simulink model "auv_backstepping2017"  (R2017b)
settings: Solver=VariableStepAuto  StartTime=0.0  StopTime=300.00  RelTol=1e-3
libraries: simulink x1
settings Model: Creator=aditya-ubuntu  LastModifiedBy=Aditya Ravi
settings SFSimCC: SimUseLocalCustomCode=on
settings RTWCC: RTWUseLocalCustomCode=on

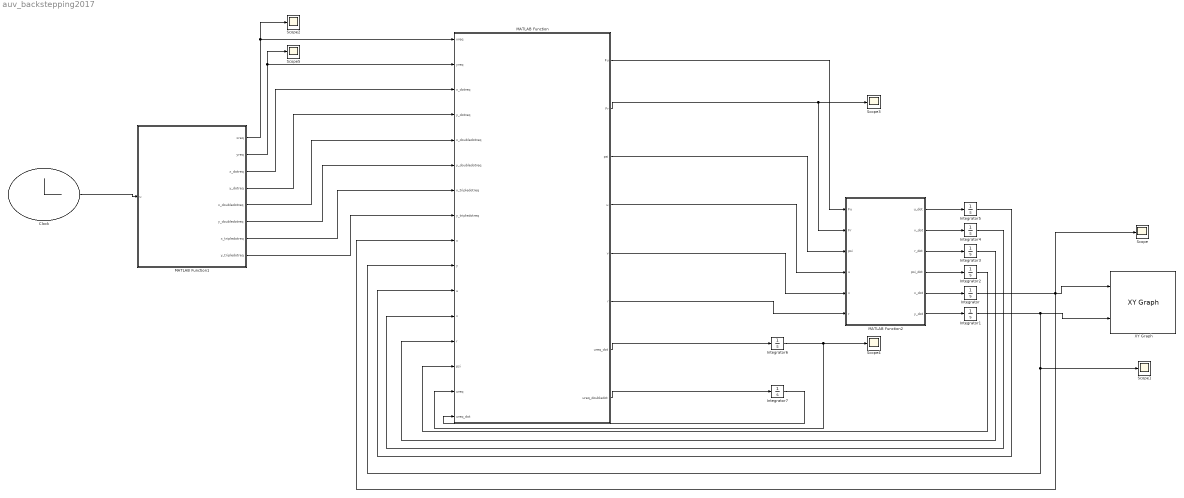
== system auv_backstepping2017 ==
  Clock : Clock
      settings: Decimation=30
  Integrator{,1..5,7} (7 alike) : Integrator
  Integrator6 : Integrator  InitialCondition=0.001  LimitOutput=on  UpperSaturationLimit=+10  LowerSaturationLimit=-10
  MATLAB Function : MATLAB Function  TreatAsAtomicUnit=on
  MATLAB Function1 : MATLAB Function  TreatAsAtomicUnit=on
  MATLAB Function2 : MATLAB Function  TreatAsAtomicUnit=on
  Scope{,1..5} (6 alike) : Scope
  XY Graph : simulink/Sinks/XY Graph  xmin=-20  xmax=20  ymin=-20  ymax=20  st=-1
  wires:
  MATLAB Function/1(Fu) -> MATLAB Function2/1(Fu)
  MATLAB Function/2(Fr) -> MATLAB Function2/2(Fr), Scope3/1
  MATLAB Function2/6(y_dot) -> Integrator1/1
  MATLAB Function2/5(x_dot) -> Integrator/1
  MATLAB Function2/4(psi_dot) -> Integrator2/1
  MATLAB Function2/3(r_dot) -> Integrator3/1
  MATLAB Function2/2(v_dot) -> Integrator4/1
  MATLAB Function2/1(u_dot) -> Integrator5/1
  Integrator/1 -> XY Graph/1, MATLAB Function/9(x), Scope/1
  Integrator1/1 -> XY Graph/2, MATLAB Function/10(y), Scope1/1
  Integrator6/1 -> MATLAB Function/15(ureq), Scope4/1
  Integrator5/1 -> MATLAB Function/11("u ")
  Integrator3/1 -> MATLAB Function/13("r ")
  Integrator2/1 -> MATLAB Function/14("psi ")
  MATLAB Function/4(u) -> MATLAB Function2/4(u)
  MATLAB Function/5(v) -> MATLAB Function2/5(v)
  MATLAB Function/6(r) -> MATLAB Function2/6(r)
  Integrator4/1 -> MATLAB Function/12("v ")
  MATLAB Function/3(psi) -> MATLAB Function2/3(psi)
  MATLAB Function/8(ureq_doubledot) -> Integrator7/1
  MATLAB Function/7(ureq_dot) -> Integrator6/1
  Integrator7/1 -> MATLAB Function/16("ureq_dot ")
  Clock/1 -> MATLAB Function1/1(u)
  MATLAB Function1/3(x_dotreq) -> MATLAB Function/3(x_dotreq)
  MATLAB Function1/4(y_dotreq) -> MATLAB Function/4(y_dotreq)
  MATLAB Function1/5(x_doubledotreq) -> MATLAB Function/5(x_doubledotreq)
  MATLAB Function1/6(y_doubledotreq) -> MATLAB Function/6(y_doubledotreq)
  MATLAB Function1/7(x_tripledotreq) -> MATLAB Function/7(x_tripledotreq)
  MATLAB Function1/8(y_tripledotreq) -> MATLAB Function/8(y_tripledotreq)
  MATLAB Function1/2(yreq) -> Scope5/1, MATLAB Function/2(yreq)
  MATLAB Function1/1(xreq) -> MATLAB Function/1(xreq), Scope2/1

== matlab function auv_backstepping2017/MATLAB Function1 ==
  data: xreq output; yreq output; u input; x_dotreq output; y_dotreq output; x_doubledotreq output; y_doubledotreq output; x_tripledotreq output; y_tripledotreq output
function [xreq,yreq,x_dotreq,y_dotreq,x_doubledotreq,y_doubledotreq,x_tripledotreq,y_tripledotreq] = fcn(u)

a = 10;
b = 0.1;

xreq = a*sin(b*u);
yreq = a*cos(b*u);

x_dotreq = a*b*cos(b*u);
y_dotreq = -a*b*sin(b*u);

x_doubledotreq = -a*b*b*sin(b*u);
y_doubledotreq = -a*b*b*cos(b*u);

x_tripledotreq = -a*b*b*b*cos(b*u);
y_tripledotreq = a*b*b*b*sin(b*u);

== matlab function auv_backstepping2017/MATLAB Function ==
  data: xreq input; yreq input; Fu output; x_dotreq input; y_dotreq input; x_doubledotreq input; y_doubledotreq input; x_tripledotreq input; y_tripledotreq input; x input; y input; u input; v input; r input; psi input; Fr output; psi output; u output; v output; r output; ureq_dot output; ureq_doubledot output; ureq input; ureq_dot input
function [Fu,Fr,psi,u,v,r,ureq_dot,ureq_doubledot] = fcn(xreq, yreq, x_dotreq, y_dotreq,x_doubledotreq,y_doubledotreq,x_tripledotreq,y_tripledotreq,x,y,u,v,r,psi,ureq,ureq_dot)

% constants 
mass= 185.0;                                                % Mass kg
Iz = 50.0;                                                  % Rotational inertia kg-m2
Xu = -30.0;                                                 % added mass kg
Yv = -90.0;                                                 % added mass kg
Nr = -30.0;                                                 % added mass kg
m = [(mass-Xu); (mass-Yv); (Iz-Nr)];                        % combined inertia and added mass terms
onebym = [1.0/(mass-Xu); 1.0/(mass-Yv); 1.0/(Iz-Nr)];       % one by combined inertia and added mass terms
d = [70.0; 100.0; 50.0];                                    % linear drag [surge, sway, yaw]

vp = sqrt(x_dotreq^2 + y_dotreq^2);
vp_dot = ((x_dotreq*x_doubledotreq)+ (y_dotreq*y_doubledotreq))/vp;
beta = atan2(y_dotreq,x_dotreq);
while(beta<0)
            beta = beta + 2*pi;
end        
while(beta>6.28)
            beta = beta - 2*pi;
end

beta_dot = ((x_dotreq*y_doubledotreq) - (y_dotreq*x_doubledotreq))/(vp^2);

if(beta_dot<=0)    
         if(ureq>=0.1)
             ureq = 0.1;
             vreq = 0;
             rreq = 0;
             psireq = beta;
             disp("ureq is equal to vp");       
         else 
             vreq = sqrt((vp*vp) - (ureq*ureq));
             mu = atan2(vreq,ureq);
             while(mu<0)
                mu = mu + 2*pi;
             end 
             while(mu>6.28)
                mu = mu - 2*pi;
             end
             psireq = beta - mu;
             rreq = beta_dot - ((ureq*vp_dot - ureq_dot*vp)/(vp*abs(vreq)));
         end 
else
         if(ureq>=0.1)
             ureq = 0.1;
             vreq = 0;
             rreq = 0;
             psireq = beta;
             disp("error");       
         else
             vreq = -sqrt((vp*vp) - (ureq*ureq));
             mu = atan2(vreq,ureq);
             while(mu<0)
                mu = mu + 2*pi;
             end    
             while(mu>6.28)
                 mu = mu - 2*pi;
             end
             psireq = beta + mu;
             rreq = beta_dot + ((ureq*vp_dot - ureq_dot*vp)/(vp*abs(vreq)));
         end 
end

beta_doubledot = ((x_dotreq*y_tripledotreq) - (y_dotreq*x_tripledotreq))/(vp^2);

if(vreq==0)
    ureq_doubledot = 0;
    rreq_dot = 0;
    ureq_dot = 0;
else 
    ureq_doubledot = -((m(1)*abs(vreq)*beta_doubledot)/(m(1)-m(2))) + ((2*d(2)*ureq_dot)/(m(1)-m(2))) + ((m(1)*beta_dot*(3*ureq*ureq - vp*vp))/((m(1)-m(2))*ureq*abs(vreq))) - ((ureq_dot^2)/(ureq));
    rreq_dot = beta_doubledot - ((vp*ureq_doubledot)/abs(vreq)) + ((vp*ureq*(ureq_dot^2))/(abs(vreq)*vreq*vreq));
    ureq_dot = ( (d(2)*vp*((ureq)^2)) - d(2)*(vp^3) - (m(1)*beta_dot*ureq*vp*abs(vreq)) + (m(1)*ureq*ureq*vp_dot) - (m(2)*vp_dot*vp*vp) )/(ureq*vp*(m(1)-m(2)));
end

fureq = (m(1)*ureq_dot)  + (d(1)*ureq) - (m(2)*vreq*rreq);
frreq = (m(3)*rreq_dot)  + (d(3)*rreq) - ((m(2)-m(1))*ureq*vreq);

% Tuning Parameters
    XYE = [ x - xreq; y - yreq ];
    ue = u - ureq;
    ve = v - vreq;
    re = r - rreq;
    psie = psi - psireq;
    
    R = [ cos(psi), -sin(psi);
            sin(psi), cos(psi)];
    
    cu = 0.5;
    k = 0.5;
    K = [k, 0;
        0, k];
    
    ku = 0.7;
    k1 = 0.7;
    K1 = [k1, 0;
        0, k1];
    
    cr = 0.1;
    c = 0.6;
    kc = 0.6;
    
    alpha_uv = - transpose(R)*(K+K1)*XYE;
    Zu = ue - alpha_uv(1);
    Zv = ve - alpha_uv(2);
    alpha_r = -cr*(-u*Zv*m(1)*onebym(2) + psie);
    Zr = re - alpha_r;
    
% Backstepping Control action 
    Tu = -(k+k1)*ue - cu*Zu - ku*Zu*(k+k1)*(k+k1);    
    Tr = -Zv - psie - cr*re*(((m(1)*u*onebym(2))^2)+1) - Zr*(c + kc*((cr*m(1)*u*onebym(2))^2));
    
% Updating Input of AUV ( Force and Torque )
    Fu = fureq + m(1)*Tu + (d(1)*ue) - m(2)*(ve*re + ve*rreq + vreq*re);      
    Fr = frreq + m(3)*Tr + (d(3)*re) + (m(2)-m(1))*(ue*ve+ ue*vreq + ureq*ve);
    
% Display 
     disp("Fureq");
     disp(fureq);
     disp("Frreq");
     disp(frreq);

%     disp("ue");
%     disp(ue);
%     disp("ve");
%     disp(ve);
%     disp("re");
%     disp(re);
%     
%     disp("Tu");
%     disp(Tu);
%     disp("Tr");
%     disp(Tr);

== matlab function auv_backstepping2017/MATLAB Function2 ==
  data: Fu input; u_dot output; Fr input; psi input; v_dot output; r_dot output; psi_dot output; x_dot output; y_dot output; u input; v input; r input
function [u_dot,v_dot,r_dot,psi_dot,x_dot,y_dot] = fcn(Fu,Fr,psi,u,v,r)

mass= 185.0;                    % Mass kg
Iz = 50.0;                      % Rotational inertia kg-m^2
Xu = -30.0;                     % added mass kg
Yv = -90.0;                     % added mass kg
Nr = -30.0;                     % added mass kg
m = [(mass-Xu),(mass-Yv), (Iz-Nr)]; % combined inertia and added mass terms
onebym = [1.0/(mass-Xu), 1.0/(mass-Yv), 1.0/(Iz-Nr)]'; % one by combined inertia and added mass terms
d = [70.0, 100.0, 50.0]';            % linear drag [surge, sway, yaw]

u_dot = ((m(2)*v*r)*onebym(1)) + ((-d(1)*u)*onebym(1)) + (Fu*onebym(1));       

v_dot = (-(m(1)*u*r)*onebym(2)) + ((-d(2)*v)*onebym(2));                          

r_dot = (((m(1)-m(2))*u*v)*onebym(3)) + ((-d(3)*r)*onebym(3)) + (Fr*onebym(3)); 

psi_dot = r;                                                                           

x_dot = (u*cos(psi)) - (v*sin(psi));                                           

y_dot = (u*sin(psi)) + (v*cos(psi));
